simulink model "kluart_5011"  (Simulink 7.8)
settings: Solver=ode4  StartTime=0.0  StopTime=inf  FixedStep=0.9  RelTol=1e-3
undefined symbols (not defined in the file): TU
libraries: serial_control_ps3510 x2, rtlab x1, serial_ps3510_recv x1, serial_send_ps3510 x1
Description:
  | Model of a simple control system for use iin training.
settings Model: Creator=Paul Baracos  LastModifiedBy=KLJS168  BufferReuse=off
settings DataIOCC: SaveOutput=off  SaveTime=off  SignalLoggingName=sigsOut
settings OptimizationCC: BlockReduction=off  BooleanDataType=off  InlineInvariantSignals=on  OptimizeBlockIOStorage=off  BufferReuse=off  ExpressionFolding=off  LocalBlockOutputs=off  InitFltsAndDblsToZero=on
settings DebuggingCC: SaveWithParameterizedLinksMsg=none  SignalResolutionControl=TryResolveAllWithWarning  SolverPrmCheckMsg=none  MultiTaskDSMMsg=warning  MultiTaskCondExecSysMsg=none  FcnCallInpInsideContextMsg=Use local settings  StrictBusMsg=None
settings HardwareCC: TargetUnknown=on
settings RTWCC: IncludeERTFirstTime=on
settings GRTTargetCC: TargetFcnLib=ansi_tfl_tmw.mat

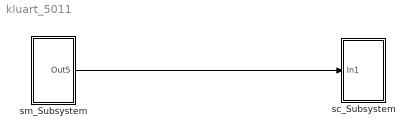
== system kluart_5011 ==
  sc_Subsystem : Subsystem
  sm_Subsystem : Subsystem
  wires:
  sm_Subsystem/1(Out5) -> sc_Subsystem/1(In1)

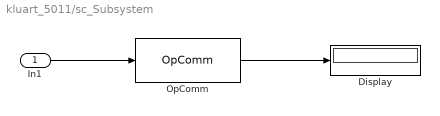
== system kluart_5011/sc_Subsystem ==
  In1 : Inport
  Display : Display
  OpComm : rtlab/OpComm  nbport=1  groupe_acq=1  subsys_rate=0  st=0  Synchronization=on  Interpolation=on  Threshold=1.0  Missed_Data=off  Sim_Time=off  Samples=off  dynSigOut=off  from_console=0  warning_done=off  writeOpCommFile=off  Offset=off
  wires:
  In1/1 -> OpComm/1
  OpComm/1 -> Display/1

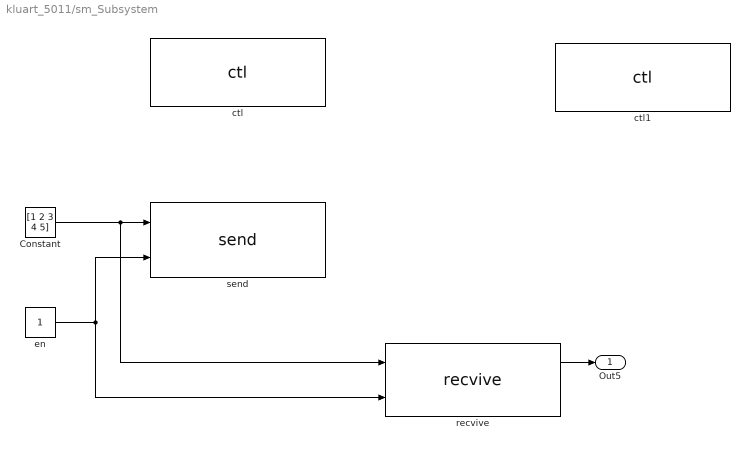
== system kluart_5011/sm_Subsystem ==
  Constant : Constant  Value=[1 2 3 4 5]
  ctl : serial_control_ps3510/ctl  choosewrongdata=TU-5011  ctlid=1  resv0=13  resv1=13  sendchl=1  resv2=Send  lenbit=Data8  paritybit=Odd  baud=9600  resv3=500000  stopbit=1  parityenbale=DIS  mode=RS485
  ctl1 : serial_control_ps3510/ctl  choosewrongdata=TU-5011  ctlid=1  resv0=13  resv1=13  sendchl=2  resv2=Receive  lenbit=Data8  paritybit=Odd  baud=9600  resv3=500000  stopbit=1  parityenbale=DIS  mode=RS485
  en : Constant
  recvive : serial_ps3510_recv/recvive  ctlid=TU-5011  resv0=13  resv1=13  recvchl=2  resv2=0  resv3=0
  send : serial_send_ps3510/send  ctlid=TU-5011  resv1=13  resv2=13  resv0=1  resv3=0
  Out5 : Outport
  wires:
  en/1 -> send/2, recvive/2
  Constant/1 -> send/1, recvive/1
  recvive/1 -> Out5/1
